simulink model "vending_machine_mealy"  (R2020b)
settings: Solver=VariableStepAuto  StartTime=0.0  StopTime=10.0  RelTol=1e-3
settings Model: Creator=Vrunda M Balgi  LastModifiedBy=Vrunda M Balgi

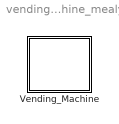
== system vending_machine_mealy ==
  Vending_Machine : Stateflow chart  TreatAsAtomicUnit=on

== stateflow chart vending_machine_mealy/Vending_Machine ==
  state Initialize
  state Select1
  state Select2
  state Select3
  state Select4
  state CheckAmount1
  state CheckAmount2
  state CheckAmount3
  state CheckAmount4
  (default) -> Initialize
  Initialize -> Select4 [order 4] : [select==4]
  Initialize -> Select1 [order 1] : [select==1]
  Initialize -> Select2 [order 2] : [select==2]
  Initialize -> Select3 [order 3] : [select==3]
  Select1 -> CheckAmount1 : [amount==10 || amount==20]
      | {money=money+amount;}
  CheckAmount1 -> Select1 : [money<30]
  Select2 -> CheckAmount2 : [amount==10 || amount==20]
      | {money=money+amount;}
  CheckAmount2 -> Select2 : [money<40]
  Select3 -> CheckAmount3 : [amount==10 || amount==20]
      | {money=money+amount;}
  CheckAmount3 -> Select3 : [money<40]
  Select4 -> CheckAmount4 : [amount==10 || amount==20]
      | {money=money+amount;}
  CheckAmount4 -> Select4 : [money<30]
